simulink model "Dragv2"  (R2022a)
settings: Solver=VariableStepAuto  StartTime=0.0  StopTime=10.0  RelTol=1e-3
model workspace (MAT data in the model file):
  A = 10
  Cd = 0.5
  FT = 1000
  k1 = 10
  rho = 1.293
undefined symbols (not defined in the file): M
settings Model: Creator=Adam Ghatta  LastModifiedBy=Adam Ghatta

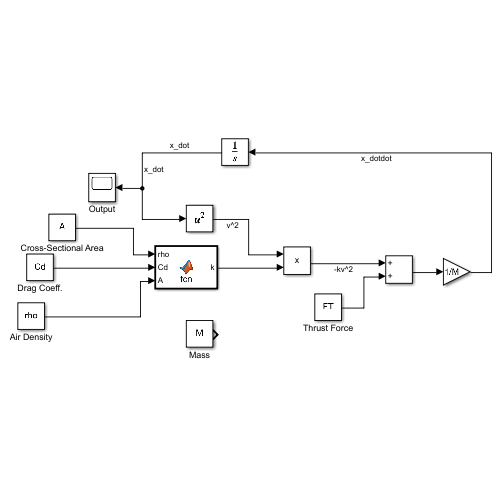
[thumbnail: Simulink's stored preview of the top-level diagram]
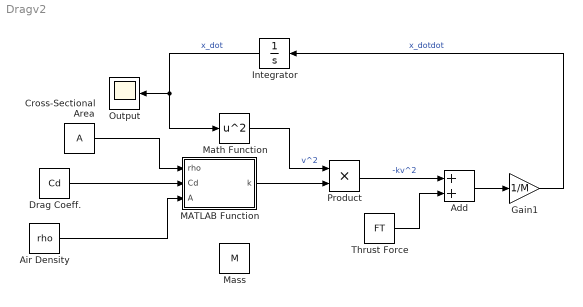
== system Dragv2 ==
  Add : Sum
  Air Density : Constant  Value=rho
  Cross-Sectional Area : Constant  Value=A
  Drag Coeff. : Constant  Value=Cd
  Gain1 : Gain  Gain=1/M
  Integrator : Integrator  InitialCondition=10
  MATLAB Function : MATLAB Function  TreatAsAtomicUnit=on
  Mass : Constant  Value=M  SampleTime=-1
  Math Function : Math  Operator=square
  Output : Scope
  Product : Product
  Thrust Force : Constant  Value=FT
  wires:
  Integrator/1 -> Math Function/1, Output/1  "x_dot"
  Gain1/1 -> Integrator/1  "x_dotdot"
  Thrust Force/1 -> Add/2
  Add/1 -> Gain1/1
  Cross-Sectional Area/1 -> MATLAB Function/1(rho)
  Drag Coeff./1 -> MATLAB Function/2(Cd)
  Air Density/1 -> MATLAB Function/3(A)
  Math Function/1 -> Product/1  "v^2"
  MATLAB Function/1(k) -> Product/2
  Product/1 -> Add/1  "-kv^2"

== matlab function Dragv2/MATLAB Function ==
  data: rho input; k output; Cd input; A input
function k = fcn(rho, Cd, A)

k = -0.5*rho*Cd*A;
